simulink model "baseline_queso"  (R2021a)
settings: Solver=FixedStepAuto  StartTime=0.0  StopTime=10.0  FixedStep=framePeriod_s  RelTol=1e-3
undefined symbols (not defined in the file or in its folder): FlightMode, framePeriod_s, Spaaro, ThrottleVelocityRange
libraries: pid_lib x14, simulink x2, sharedtransform x1
(part 1 of 2)
settings Model: Creator=brian  LastModifiedBy=vaughnweirens
settings SolverCC: AlgebraicLoopSolver=TrustRegion
settings OptimizationCC: DefaultParameterBehavior=Inlined  GainParamInheritBuiltInType=on  UseFloatMulNetSlope=on  DefaultUnderspecifiedDataType=single  InlineInvariantSignals=on  PassReuseOutputArgsAs=Individual arguments  ZeroExternalMemoryAtStartup=off  ZeroInternalMemoryAtStartup=off  NoFixptDivByZeroProtection=on  EfficientFloat2IntCast=on  LifeSpan=1  OptimizeBlockOrder=speed  DifferentSizesBufferReuse=on  EfficientTunableParamExpr=on
settings DebuggingCC: ParameterTunabilityLossMsg=error  SFMachineParentedDataDiag=warning
settings HardwareCC: ProdBitPerPointer=32  ProdBitPerSizeT=32  ProdBitPerPtrDiffT=32  ProdLargestAtomicInteger=Long  ProdLargestAtomicFloat=Double  ProdWordSize=32  ProdLongLongMode=on  ProdHWDeviceType=NXP->Cortex-M4
settings ModelReferenceCC: ModelReferenceNumInstancesAllowed=Single
settings SFSimCC: SimParseCustomCode=off  MATLABDynamicMemAlloc=off
settings RTWCC: SystemTargetFile=ert.tlc  GenCodeOnly=on  TemplateMakefile=ert_default_tmf  RTWVerbose=off  Toolchain=Microsoft Visual C++ 2019 v16.0 | nmake (64-bit Windows)  BuildConfiguration=Faster Runs  TargetLang=C++
settings CodeAppCC: ForceParamTrailComments=on  IgnoreCustomStorageClasses=off  OperatorAnnotations=on  SimulinkDataObjDesc=on  SFDataObjDesc=on  CustomSymbolStrGlobalVar=rt$N$M  CustomSymbolStrType=$N$M  CustomSymbolStrFcn=$N$M$F  CustomSymbolStrMacro=$N$M  InsertBlockDesc=on
settings ERTTargetCC: TargetLangStandard=C++03 (ISO)  IncludeMdlTerminateFcn=off  CombineSignalStateStructs=on  SuppressErrorStatus=on  SupportAbsoluteTime=off  CodeInterfacePackaging=C++ class  SupportNonFinite=off  SupportComplex=off  ERTHeaderFileRootName=autocode$E  ERTSourceFileRootName=autocode$E  InlinedParameterPlacement=NonHierarchical  RootIOFormat=Structure reference  ERTCustomFileTemplate=example_file_process.tlc  ERTFilePackagingFormat=Compact  ArrayContainerType=std::array

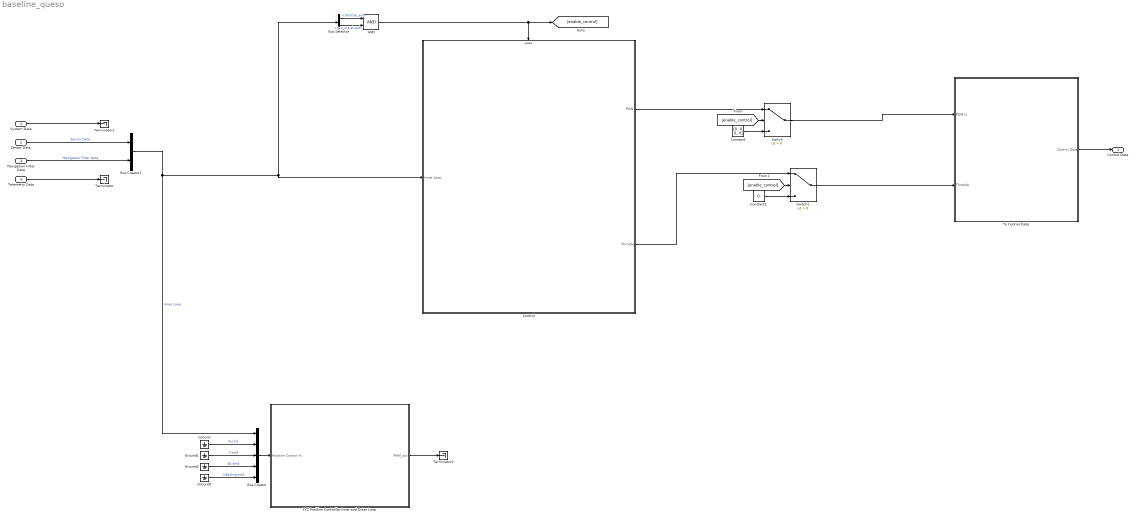
== system baseline_queso ==
  System Data : Inport  OutDataTypeStr=Bus: SysData  SampleTime=framePeriod_s  BusOutputAsStruct=on
  Sensor Data : Inport  Port=2  OutDataTypeStr=Bus: SensorData  SampleTime=framePeriod_s  BusOutputAsStruct=on
  Navigation Filter Data : Inport  Port=3  OutDataTypeStr=Bus: NavData  SampleTime=framePeriod_s  BusOutputAsStruct=on
  Telemetry Data : Inport  Port=4  OutDataTypeStr=Bus: TelemData  SampleTime=framePeriod_s  BusOutputAsStruct=on
  AND : Logic  IconShape=distinctive  AllPortsSameDT=off  OutDataTypeStr=boolean
  Bus Creator : BusCreator  Inputs=5
  Bus Creator1 : BusCreator  Inputs=2
  Bus Selector : BusSelector  OutputSignals=Sensor Data.inceptor.throttle_en,Navigation Filter Data.nav_initialized
  Constant : Constant  Value=[0, 0, 0, 0]  SampleTime=framePeriod_s
  Constant1 : Constant  Value=0  SampleTime=framePeriod_s
  Control : Subsystem
  Ground{,1..3} (4 alike) : Ground
  Switch : Switch  Criteria=u2 > Threshold
  Switch1 : Switch  Criteria=u2 > Threshold
  Terminator : Terminator
  Terminator1 : Terminator
  Terminator2 : Terminator
  To Control Data : Subsystem
  XYZ Position Controller Inner and Outer Loop : Subsystem
  Control Data : Outport  OutDataTypeStr=Bus: ControlData  SampleTime=framePeriod_s  BusOutputAsStruct=on
  wires:
  Telemetry Data/1 -> Terminator/1
  System Data/1 -> Terminator1/1
  Sensor Data/1 -> Bus Creator1/1  "Sensor Data"
  Navigation Filter Data/1 -> Bus Creator1/2  "Navigation Filter Data"
  Bus Creator1/1 -> Bus Creator/1, Bus Selector/1, Control/1(Inner Loop)  "Inner Loop"
  To Control Data/1(Control Data) -> Control Data/1
  Ground1/1 -> Bus Creator/3  "Y-cmd"
  Ground/1 -> Bus Creator/2  "X-cmd"
  Ground3/1 -> Bus Creator/5  "Heading-cmd"
  Ground2/1 -> Bus Creator/4  "Alt-cmd"
  Bus Creator/1 -> XYZ Position Controller Inner and Outer Loop/1(Position Control In)
  XYZ Position Controller Inner and Outer Loop/1(PWM_out) -> Terminator2/1
  Bus Selector/1 -> AND/1  "<throttle_en>"
  Bus Selector/2 -> AND/2  "<nav_initialized>"
  AND/1 -> [enable_control], Control/Enable
  [enable_control] -> Switch/2
  Constant/1 -> Switch/3
  Constant1/1 -> Switch1/3
  [enable_control] -> Switch1/2
  Control/1(PWM) -> Switch/1
  Control/2("Throttle ") -> Switch1/1
  Switch1/1 -> To Control Data/2("Throttle ")
  Switch/1 -> To Control Data/1(PWM In)

== system baseline_queso/Control ==
  Inner Loop : Inport
  Enable : EnablePort  PropagateVarSize=During execution
  Bus Creator4 : BusCreator  Inputs=4
  Inner Loop Control : Subsystem
  Motor Mixing Algorithm : Subsystem
  Outer Loop Control : Subsystem
  PWM : Outport
  "Throttle " : Outport  Port=2
  wires:
  Outer Loop Control/1("Throttle ") -> "Throttle "/1, Bus Creator4/1
  Motor Mixing Algorithm/1(PWM) -> PWM/1
  Inner Loop/1 -> Inner Loop Control/1(Inner Loop), Outer Loop Control/1(Outer Loop In)
  Inner Loop Control/3(Yaw) -> Bus Creator4/4
  Inner Loop Control/1(Roll) -> Bus Creator4/2
  Inner Loop Control/2(Pitch) -> Bus Creator4/3
  Bus Creator4/1 -> Motor Mixing Algorithm/1(MMA Bus)

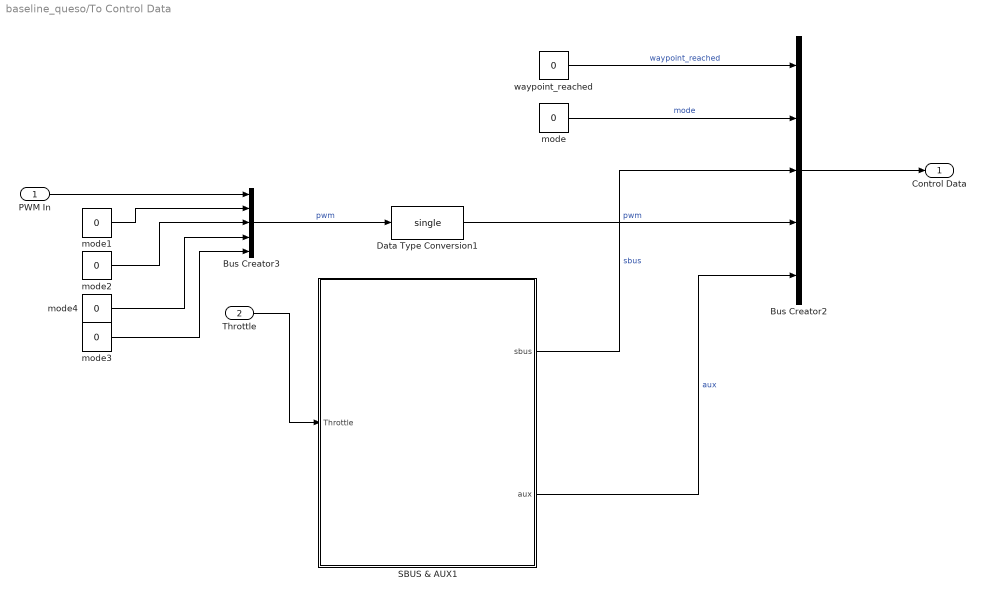
== system baseline_queso/To Control Data ==
  PWM In : Inport
  "Throttle " : Inport  Port=2
  Bus Creator2 : BusCreator  Inputs=5  OutDataTypeStr=Bus: ControlData  NonVirtualBus=on
  Bus Creator3 : BusCreator  Inputs=5
  Data Type Conversion1 : DataTypeConversion  OutDataTypeStr=single
  SBUS & AUX1 : Subsystem
  mode{,1..4} (5 alike) : Constant  Value=0  OutDataTypeStr=int8  SampleTime=framePeriod_s
  waypoint_reached : Constant  Value=0  OutDataTypeStr=boolean  SampleTime=framePeriod_s
  Control Data : Outport  OutDataTypeStr=Bus: ControlData  SampleTime=framePeriod_s  BusOutputAsStruct=on
  wires:
  waypoint_reached/1 -> Bus Creator2/1  "waypoint_reached"
  Bus Creator3/1 -> Data Type Conversion1/1  "pwm"
  mode/1 -> Bus Creator2/2  "mode"
  Bus Creator2/1 -> Control Data/1
  SBUS & AUX1/1(sbus) -> Bus Creator2/3  "sbus"
  SBUS & AUX1/2(aux) -> Bus Creator2/5  "aux"
  Data Type Conversion1/1 -> Bus Creator2/4  "pwm"
  PWM In/1 -> Bus Creator3/1
  "Throttle "/1 -> SBUS & AUX1/1("Throttle ")
  mode1/1 -> Bus Creator3/2
  mode2/1 -> Bus Creator3/3
  mode4/1 -> Bus Creator3/4
  mode3/1 -> Bus Creator3/5

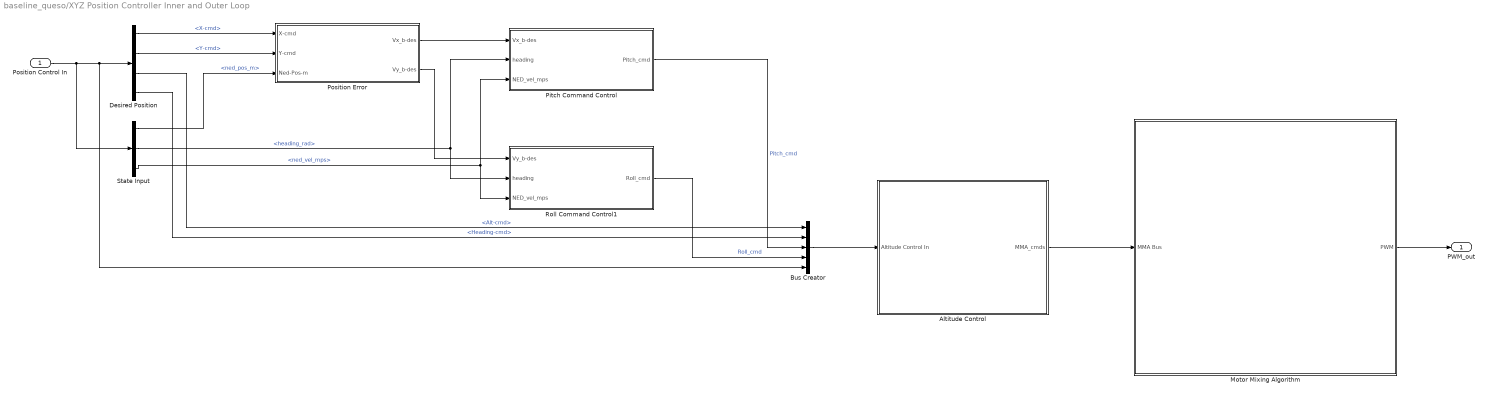
== system baseline_queso/XYZ Position Controller Inner and Outer Loop ==
  Position Control In : Inport
  Altitude Control : Subsystem
  Bus Creator : BusCreator  Inputs=5
  Desired Position : BusSelector  OutputSignals=X-cmd,Y-cmd,Alt-cmd,Heading-cmd
  Motor Mixing Algorithm : Subsystem
  Pitch Command Control : Subsystem
  Position Error : Subsystem
  Roll Command Control1 : Subsystem
  State Input : BusSelector  OutputSignals=Inner Loop.Navigation Filter Data.ned_pos_m,Inner Loop.Navigation Filter Data.heading_rad,Inner Loop.Navigation Filter Data.ned_vel_mps
  PWM_out : Outport
  wires:
  Position Control In/1 -> State Input/1, Bus Creator/5, Desired Position/1
  Desired Position/1 -> Position Error/1(X-cmd)  "<X-cmd>"
  Desired Position/2 -> Position Error/2(Y-cmd)  "<Y-cmd>"
  State Input/1 -> Position Error/3(Ned-Pos-m)  "<ned_pos_m>"
  Position Error/1(Vx_b-des) -> Pitch Command Control/1(Vx_b-des)
  State Input/3 -> Roll Command Control1/3(NED_vel_mps), Pitch Command Control/3(NED_vel_mps)  "<ned_vel_mps>"
  State Input/2 -> Pitch Command Control/2(heading), Roll Command Control1/2(heading)  "<heading_rad>"
  Position Error/2(Vy_b-des) -> Roll Command Control1/1(Vy_b-des)
  Bus Creator/1 -> Altitude Control/1(Altitude Control In)
  Desired Position/3 -> Bus Creator/1  "<Alt-cmd>"
  Desired Position/4 -> Bus Creator/2  "<Heading-cmd>"
  Pitch Command Control/1(Pitch_cmd) -> Bus Creator/3  "Pitch_cmd"
  Roll Command Control1/1(Roll_cmd) -> Bus Creator/4  "Roll_cmd"
  Altitude Control/1(MMA_cmds) -> Motor Mixing Algorithm/1(MMA Bus)
  Motor Mixing Algorithm/1(PWM) -> PWM_out/1

== system baseline_queso/Control/Inner Loop Control ==
  Inner Loop : Inport
  Pitch Controller : Subsystem
  Roll Controller : Subsystem
  Yaw Rate Controller : Subsystem
  Roll : Outport
  Pitch : Outport  Port=2
  Yaw : Outport  Port=3
  wires:
  Inner Loop/1 -> Yaw Rate Controller/1(Yaw Bus), Roll Controller/1(Roll Bus), Pitch Controller/1(Pitch Bus)
  Roll Controller/1(roll_cc) -> Roll/1  "roll_cc"
  Pitch Controller/1(pitch_cc) -> Pitch/1  "pitch_cc"
  Yaw Rate Controller/1(yaw_cc) -> Yaw/1  "yaw_cc"

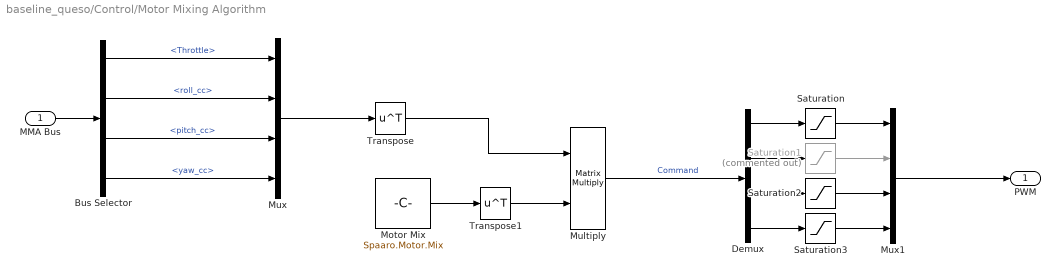
== system baseline_queso/Control/Motor Mixing Algorithm ==
  MMA Bus : Inport
  Bus Selector : BusSelector  OutputSignals=Throttle,roll_cc,pitch_cc,yaw_cc
  Demux : Demux
  Motor Mix : Constant  Value=Spaaro.Motor.Mix  OutDataTypeStr=single
  Multiply : Product  Inputs=**  Multiplication=Matrix(*)
  Mux : Mux
  Mux1 : Mux
  Saturation : Saturate  UpperLimit=1  LowerLimit=0
  Saturation1 : Saturate  Commented=on  UpperLimit=1  LowerLimit=0
  Saturation2 : Saturate  UpperLimit=1  LowerLimit=0
  Saturation3 : Saturate  UpperLimit=1  LowerLimit=0
  Transpose : Math  Operator=transpose  SaturateOnIntegerOverflow=on
  Transpose1 : Math  Operator=transpose  SaturateOnIntegerOverflow=on
  PWM : Outport
  wires:
  Mux/1 -> Transpose/1
  Transpose/1 -> Multiply/1
  Multiply/1 -> Demux/1  "Command"
  Saturation/1 -> Mux1/1
  Saturation1/1 -> Mux1/2
  Saturation2/1 -> Mux1/3
  Saturation3/1 -> Mux1/4
  Mux1/1 -> PWM/1
  Demux/1 -> Saturation/1
  Demux/2 -> Saturation1/1
  Demux/3 -> Saturation2/1
  Demux/4 -> Saturation3/1
  Motor Mix/1 -> Transpose1/1
  Transpose1/1 -> Multiply/2
  MMA Bus/1 -> Bus Selector/1
  Bus Selector/1 -> Mux/1  "<Throttle>"
  Bus Selector/2 -> Mux/2  "<roll_cc>"
  Bus Selector/3 -> Mux/3  "<pitch_cc>"
  Bus Selector/4 -> Mux/4  "<yaw_cc>"

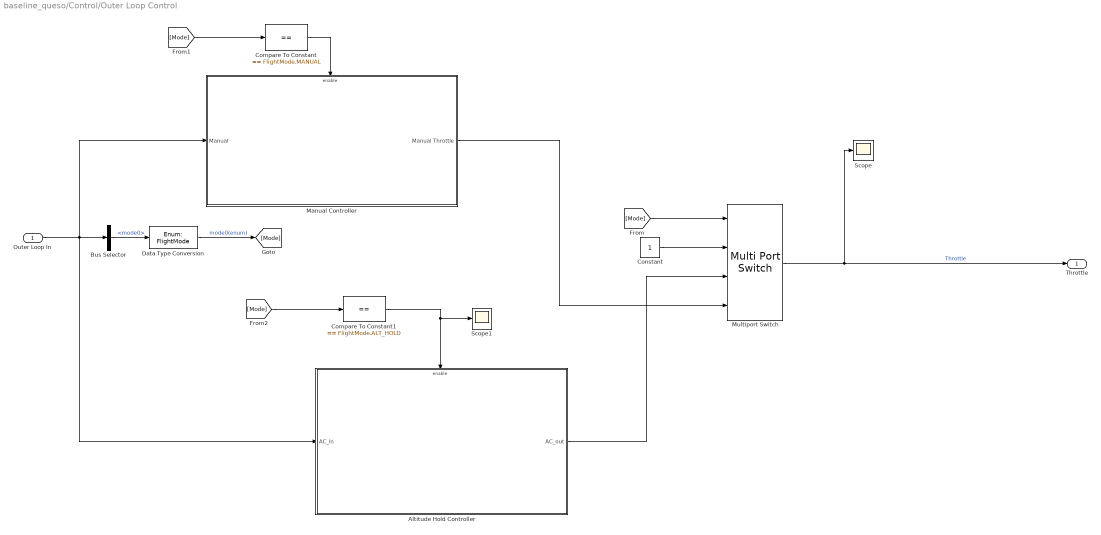
== system baseline_queso/Control/Outer Loop Control ==
  Outer Loop In : Inport
  Altitude Hold Controller : Subsystem
  Bus Selector : BusSelector  OutputSignals=Sensor Data.inceptor.mode0
  Compare To Constant : simulink/Logic and Bit Operations/Compare To Constant  relop===  const=FlightMode.MANUAL  OutDataTypeStr=boolean
  Compare To Constant1 : simulink/Logic and Bit Operations/Compare To Constant  relop===  const=FlightMode.ALT_HOLD  OutDataTypeStr=boolean
  Constant : Constant
  Data Type Conversion : DataTypeConversion  OutDataTypeStr=Enum: FlightMode
  Manual Controller : Subsystem
  Multiport Switch : MultiPortSwitch  DataPortOrder=Specify indices  DataPortIndices={FlightMode.AUTO, FlightMode.ALT_HOLD, FlightMode.MANUAL}
  Scope : Scope
  Scope1 : Scope
  "Throttle " : Outport
  wires:
  Multiport Switch/1 -> Scope/1, "Throttle "/1  "Throttle"
  [Mode] -> Compare To Constant/1
  Compare To Constant1/1 -> Scope1/1, Altitude Hold Controller/Enable
  Altitude Hold Controller/1(AC_out) -> Multiport Switch/3
  Compare To Constant/1 -> Manual Controller/Enable
  Data Type Conversion/1 -> [Mode]  "mode0(enum)"
  [Mode] -> Compare To Constant1/1
  [Mode] -> Multiport Switch/1
  Bus Selector/1 -> Data Type Conversion/1  "<mode0>"
  Outer Loop In/1 -> Altitude Hold Controller/1(AC_in), Bus Selector/1, Manual Controller/1(Manual)
  Constant/1 -> Multiport Switch/2
  Manual Controller/1(Manual Throttle) -> Multiport Switch/4

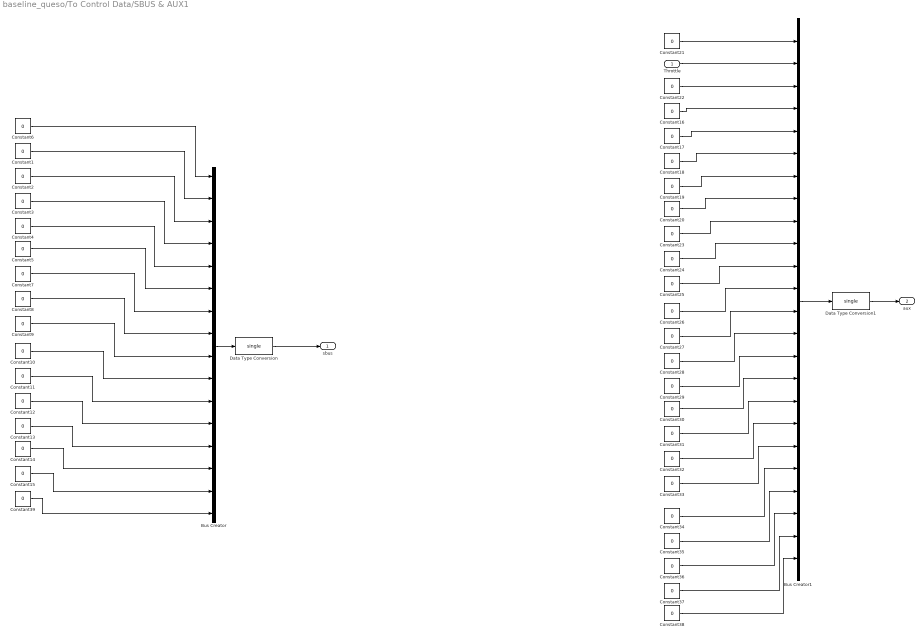
== system baseline_queso/To Control Data/SBUS & AUX1 ==
  "Throttle " : Inport
  Bus Creator : BusCreator  Inputs=16
  Bus Creator1 : BusCreator  Inputs=24
  Constant{1..39} (39 alike) : Constant  Value=0  OutDataTypeStr=single  SampleTime=framePeriod_s
  Data Type Conversion : DataTypeConversion  OutDataTypeStr=single
  Data Type Conversion1 : DataTypeConversion  OutDataTypeStr=single
  sbus : Outport  SampleTime=framePeriod_s
  aux : Outport  Port=2
  wires:
  Bus Creator/1 -> Data Type Conversion/1
  Data Type Conversion/1 -> sbus/1
  Bus Creator1/1 -> Data Type Conversion1/1
  Data Type Conversion1/1 -> aux/1
  Constant21/1 -> Bus Creator1/1
  "Throttle "/1 -> Bus Creator1/2
  Constant22/1 -> Bus Creator1/3
  Constant16/1 -> Bus Creator1/4
  Constant17/1 -> Bus Creator1/5
  Constant18/1 -> Bus Creator1/6
  Constant19/1 -> Bus Creator1/7
  Constant20/1 -> Bus Creator1/8
  Constant23/1 -> Bus Creator1/9
  Constant24/1 -> Bus Creator1/10
  Constant25/1 -> Bus Creator1/11
  Constant26/1 -> Bus Creator1/12
  Constant27/1 -> Bus Creator1/13
  Constant28/1 -> Bus Creator1/14
  Constant29/1 -> Bus Creator1/15
  Constant30/1 -> Bus Creator1/16
  Constant31/1 -> Bus Creator1/17
  Constant32/1 -> Bus Creator1/18
  Constant33/1 -> Bus Creator1/19
  Constant34/1 -> Bus Creator1/20
  Constant35/1 -> Bus Creator1/21
  Constant36/1 -> Bus Creator1/22
  Constant37/1 -> Bus Creator1/23
  Constant38/1 -> Bus Creator1/24
  Constant12/1 -> Bus Creator/12
  Constant11/1 -> Bus Creator/11
  Constant10/1 -> Bus Creator/10
  Constant9/1 -> Bus Creator/9
  Constant8/1 -> Bus Creator/8
  Constant7/1 -> Bus Creator/7
  Constant4/1 -> Bus Creator/5
  Constant5/1 -> Bus Creator/6
  Constant3/1 -> Bus Creator/4
  Constant2/1 -> Bus Creator/3
  Constant1/1 -> Bus Creator/2
  Constant6/1 -> Bus Creator/1
  Constant39/1 -> Bus Creator/16
  Constant15/1 -> Bus Creator/15
  Constant13/1 -> Bus Creator/13
  Constant14/1 -> Bus Creator/14

== system baseline_queso/XYZ Position Controller Inner and Outer Loop/Altitude Control ==
  Altitude Control In : Inport
  Bus Creator : BusCreator  Inputs=4
  Pitch Control : Subsystem
  Roll Control : Subsystem
  Throttle Control : Subsystem
  Yaw Control : Subsystem
  MMA_cmds : Outport
  wires:
  Altitude Control In/1 -> Throttle Control/1(Altitude Control In), Roll Control/1(Roll Control In), Pitch Control/1(Pitch Control In), Yaw Control/1(Yaw Control In)
  Bus Creator/1 -> MMA_cmds/1
  Throttle Control/1(Throttle_des) -> Bus Creator/1  "Throttle_des"
  Roll Control/1(Roll_cntrl) -> Bus Creator/2  "Roll_cntrl"
  Pitch Control/1(Pitch_cntrl) -> Bus Creator/3  "Pitch_cntrl"
  Yaw Control/1(Yaw_cntl) -> Bus Creator/4  "Yaw_cntrl"

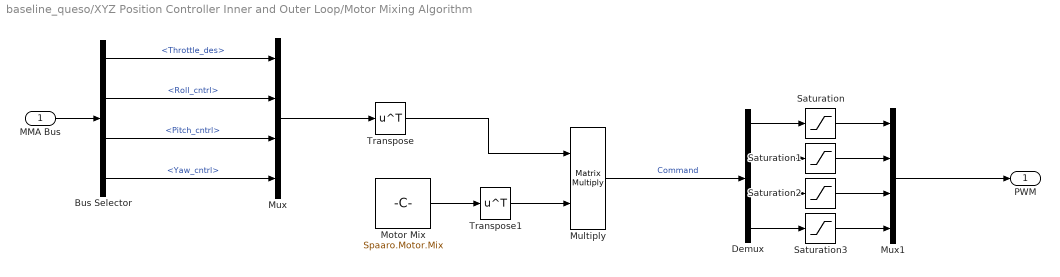
== system baseline_queso/XYZ Position Controller Inner and Outer Loop/Motor Mixing Algorithm ==
  MMA Bus : Inport
  Bus Selector : BusSelector  OutputSignals=Throttle_des,Roll_cntrl,Pitch_cntrl,Yaw_cntrl
  Demux : Demux
  Motor Mix : Constant  Value=Spaaro.Motor.Mix  OutDataTypeStr=single
  Multiply : Product  Inputs=**  Multiplication=Matrix(*)
  Mux : Mux
  Mux1 : Mux
  Saturation{,1..3} (4 alike) : Saturate  UpperLimit=1  LowerLimit=0
  Transpose : Math  Operator=transpose  SaturateOnIntegerOverflow=on
  Transpose1 : Math  Operator=transpose  SaturateOnIntegerOverflow=on
  PWM : Outport
  wires:
  Mux/1 -> Transpose/1
  Transpose/1 -> Multiply/1
  Multiply/1 -> Demux/1  "Command"
  Saturation/1 -> Mux1/1
  Saturation1/1 -> Mux1/2
  Saturation2/1 -> Mux1/3
  Saturation3/1 -> Mux1/4
  Mux1/1 -> PWM/1
  Demux/1 -> Saturation/1
  Demux/2 -> Saturation1/1
  Demux/3 -> Saturation2/1
  Demux/4 -> Saturation3/1
  Motor Mix/1 -> Transpose1/1
  Transpose1/1 -> Multiply/2
  MMA Bus/1 -> Bus Selector/1
  Bus Selector/1 -> Mux/1  "<Throttle_des>"
  Bus Selector/2 -> Mux/2  "<Roll_cntrl>"
  Bus Selector/3 -> Mux/3  "<Pitch_cntrl>"
  Bus Selector/4 -> Mux/4  "<Yaw_cntrl>"

== system baseline_queso/XYZ Position Controller Inner and Outer Loop/Pitch Command Control ==
  Vx_b-des : Inport
  heading : Inport  Port=2
  NED_vel_mps : Inport  Port=3
  Cos : Trigonometry  Operator=cos
  Divide : Product  Inputs=**
  PID Controller : pid_lib/PID Controller  Controller=PID  Form=Parallel  TimeDomain=Discrete-time  UseExternalTs=off  SampleTime=-1  IntegratorMethod=Forward Euler  FilterMethod=Forward Euler  ControllerParametersSource=internal  P=1  I=1  D=0  UseFilter=on  N=100  TunerSelectOption=Transfer Function Based (PID Tuner App)  InitialConditionSource=internal  InitialConditionForIntegrator=0  InitialConditionForFilter=0  DifferentiatorICPrevScaledInput=0  ExternalReset=none  TrackingMode=off  Kt=1  LimitOutput=off  SatLimitsSource=internal  UpperSaturationLimit=inf  LowerSaturationLimit=-inf  LinearizeAsGain=on  AntiWindupMode=none  Kb=1  POutMin=[]  POutMax=[]  IOutMin=[]  IOutMax=[]  DOutMin=[]  DOutMax=[]  NOutMin=[]  NOutMax=[]  SumOutMin=[]  SumOutMax=[]  SaturationOutMin=[]  SaturationOutMax=[]  PParamMin=[]  PParamMax=[]  IParamMin=[]  IParamMax=[]  DParamMin=[]  DParamMax=[]  NParamMin=[]  NParamMax=[]  KbParamMin=[]  KbParamMax=[]  KtParamMin=[]  KtParamMax=[]  KbOutMin=[]  KbOutMax=[]  KtOutMin=[]  KtOutMax=[]  IntegratorOutMin=[]  IntegratorOutMax=[]  FilterOutMin=[]  FilterOutMax=[]  SumI1OutMin=[]  SumI1OutMax=[]  SumI2OutMin=[]  SumI2OutMax=[]  SumI3OutMin=[]  SumI3OutMax=[]  SumI4OutMin=[]  SumI4OutMax=[]  SumDOutMin=[]  SumDOutMax=[]  DifferentiatorOutMin=[]  DifferentiatorOutMax=[]  FilterDiffOutCoefMin=[]  FilterDiffOutCoefMax=[]  ReciprocalOutMin=[]  ReciprocalOutMax=[]  SumDenOutMin=[]  SumDenOutMax=[]  SumNumOutMin=[]  SumNumOutMax=[]  DivideOutMin=[]  DivideOutMax=[]  UdiffTsProdOutMin=[]  UdiffTsProdOutMax=[]  NTsProdOutMin=[]  NTsProdOutMax=[]  UintegralTsProdOutMin=[]  UintegralTsProdOutMax=[]  UngainTsProdOutMin=[]  UngainTsProdOutMax=[]  IntegratorContinuousStateAttributes=''  IntegratorStateMustResolveToSignalObject=off  IntegratorRTWStateStorageClass=Auto  FilterContinuousStateAttributes=''  FilterStateMustResolveToSignalObject=off  FilterRTWStateStorageClass=Auto  ParallelPVariant=InternalParameters  IdealPVariant=Disabled  IVariant=InternalParameters  DVariant=InternalParameters  IntegratorVariant=Discrete  SatVariant=Disabled  AWVariant=Passthrough  PCopyVariant=Disabled  TRVariant=Disabled  FdbkBlocksVariant=Forward  IdealPFdbkVariant=Disabled  SatFdbkVariant=Disabled  DerivativeFilterVariant=ForwardEulerFilter  NVariant=InternalParameters  NCopyVariant=Disabled  FilterICVariant=InternalICsFilter  IntegratorICVariant=InternalICs  ExternalResetVariant=Disabled  TRSumVariant=Passthrough  SumFdbkVariant=Disabled  SumVariant=Sum_PID  TsampFilterVariant=InternalTs  TsampNgainVariant=Passthrough  TsampIntegralVariant=Passthrough  ExternalSaturationOutDataTypeStr=Inherit: Same as second input
  Selector : Selector  InputPortWidth=3  IndexOptions=Index vector (dialog)  Indices=[1]  OutputSizes=1
  Sum : Sum  Inputs=|+-
  Pitch_cmd : Outport
  wires:
  Vx_b-des/1 -> Sum/1
  heading/1 -> Cos/1
  NED_vel_mps/1 -> Selector/1
  Cos/1 -> Divide/1
  Selector/1 -> Divide/2
  Divide/1 -> Sum/2
  Sum/1 -> PID Controller/1
  PID Controller/1 -> Pitch_cmd/1

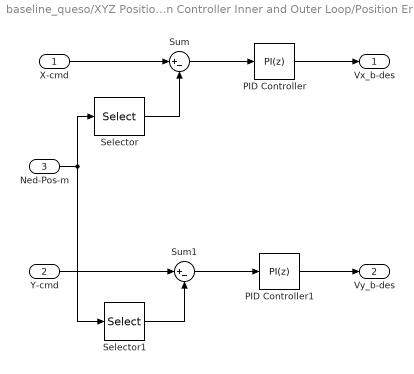
== system baseline_queso/XYZ Position Controller Inner and Outer Loop/Position Error ==
  X-cmd : Inport
  Y-cmd : Inport  Port=2
  Ned-Pos-m : Inport  Port=3
  PID Controller : pid_lib/PID Controller  Controller=PI  Form=Parallel  TimeDomain=Discrete-time  UseExternalTs=off  SampleTime=-1  IntegratorMethod=Forward Euler  FilterMethod=Forward Euler  ControllerParametersSource=internal  P=1  I=1  D=0  UseFilter=on  N=100  TunerSelectOption=Transfer Function Based (PID Tuner App)  InitialConditionSource=internal  InitialConditionForIntegrator=0  InitialConditionForFilter=0  DifferentiatorICPrevScaledInput=0  ExternalReset=none  TrackingMode=off  Kt=1  LimitOutput=off  SatLimitsSource=internal  UpperSaturationLimit=inf  LowerSaturationLimit=-inf  LinearizeAsGain=on  AntiWindupMode=none  Kb=1  POutMin=[]  POutMax=[]  IOutMin=[]  IOutMax=[]  DOutMin=[]  DOutMax=[]  NOutMin=[]  NOutMax=[]  SumOutMin=[]  SumOutMax=[]  SaturationOutMin=[]  SaturationOutMax=[]  PParamMin=[]  PParamMax=[]  IParamMin=[]  IParamMax=[]  DParamMin=[]  DParamMax=[]  NParamMin=[]  NParamMax=[]  KbParamMin=[]  KbParamMax=[]  KtParamMin=[]  KtParamMax=[]  KbOutMin=[]  KbOutMax=[]  KtOutMin=[]  KtOutMax=[]  IntegratorOutMin=[]  IntegratorOutMax=[]  FilterOutMin=[]  FilterOutMax=[]  SumI1OutMin=[]  SumI1OutMax=[]  SumI2OutMin=[]  SumI2OutMax=[]  SumI3OutMin=[]  SumI3OutMax=[]  SumI4OutMin=[]  SumI4OutMax=[]  SumDOutMin=[]  SumDOutMax=[]  DifferentiatorOutMin=[]  DifferentiatorOutMax=[]  FilterDiffOutCoefMin=[]  FilterDiffOutCoefMax=[]  ReciprocalOutMin=[]  ReciprocalOutMax=[]  SumDenOutMin=[]  SumDenOutMax=[]  SumNumOutMin=[]  SumNumOutMax=[]  DivideOutMin=[]  DivideOutMax=[]  UdiffTsProdOutMin=[]  UdiffTsProdOutMax=[]  NTsProdOutMin=[]  NTsProdOutMax=[]  UintegralTsProdOutMin=[]  UintegralTsProdOutMax=[]  UngainTsProdOutMin=[]  UngainTsProdOutMax=[]  IntegratorContinuousStateAttributes=''  IntegratorStateMustResolveToSignalObject=off  IntegratorRTWStateStorageClass=Auto  FilterContinuousStateAttributes=''  FilterStateMustResolveToSignalObject=off  FilterRTWStateStorageClass=Auto  ParallelPVariant=InternalParameters  IdealPVariant=Disabled  IVariant=InternalParameters  DVariant=Disabled  IntegratorVariant=Discrete  SatVariant=Disabled  AWVariant=Passthrough  PCopyVariant=Disabled  TRVariant=Disabled  FdbkBlocksVariant=Forward  IdealPFdbkVariant=Disabled  SatFdbkVariant=Disabled  DerivativeFilterVariant=Disabled  NVariant=Disabled  NCopyVariant=Disabled_SignalSpec  FilterICVariant=Disabled  IntegratorICVariant=InternalICs  ExternalResetVariant=Disabled  TRSumVariant=Passthrough  SumFdbkVariant=Disabled  SumVariant=Sum_PI  TsampFilterVariant=InternalTs  TsampNgainVariant=Passthrough  TsampIntegralVariant=Passthrough  ExternalSaturationOutDataTypeStr=Inherit: Same as second input
  PID Controller1 : pid_lib/PID Controller  Controller=PI  Form=Parallel  TimeDomain=Discrete-time  UseExternalTs=off  SampleTime=-1  IntegratorMethod=Forward Euler  FilterMethod=Forward Euler  ControllerParametersSource=internal  P=1  I=1  D=0  UseFilter=on  N=100  TunerSelectOption=Transfer Function Based (PID Tuner App)  InitialConditionSource=internal  InitialConditionForIntegrator=0  InitialConditionForFilter=0  DifferentiatorICPrevScaledInput=0  ExternalReset=none  TrackingMode=off  Kt=1  LimitOutput=off  SatLimitsSource=internal  UpperSaturationLimit=inf  LowerSaturationLimit=-inf  LinearizeAsGain=on  AntiWindupMode=none  Kb=1  POutMin=[]  POutMax=[]  IOutMin=[]  IOutMax=[]  DOutMin=[]  DOutMax=[]  NOutMin=[]  NOutMax=[]  SumOutMin=[]  SumOutMax=[]  SaturationOutMin=[]  SaturationOutMax=[]  PParamMin=[]  PParamMax=[]  IParamMin=[]  IParamMax=[]  DParamMin=[]  DParamMax=[]  NParamMin=[]  NParamMax=[]  KbParamMin=[]  KbParamMax=[]  KtParamMin=[]  KtParamMax=[]  KbOutMin=[]  KbOutMax=[]  KtOutMin=[]  KtOutMax=[]  IntegratorOutMin=[]  IntegratorOutMax=[]  FilterOutMin=[]  FilterOutMax=[]  SumI1OutMin=[]  SumI1OutMax=[]  SumI2OutMin=[]  SumI2OutMax=[]  SumI3OutMin=[]  SumI3OutMax=[]  SumI4OutMin=[]  SumI4OutMax=[]  SumDOutMin=[]  SumDOutMax=[]  DifferentiatorOutMin=[]  DifferentiatorOutMax=[]  FilterDiffOutCoefMin=[]  FilterDiffOutCoefMax=[]  ReciprocalOutMin=[]  ReciprocalOutMax=[]  SumDenOutMin=[]  SumDenOutMax=[]  SumNumOutMin=[]  SumNumOutMax=[]  DivideOutMin=[]  DivideOutMax=[]  UdiffTsProdOutMin=[]  UdiffTsProdOutMax=[]  NTsProdOutMin=[]  NTsProdOutMax=[]  UintegralTsProdOutMin=[]  UintegralTsProdOutMax=[]  UngainTsProdOutMin=[]  UngainTsProdOutMax=[]  IntegratorContinuousStateAttributes=''  IntegratorStateMustResolveToSignalObject=off  IntegratorRTWStateStorageClass=Auto  FilterContinuousStateAttributes=''  FilterStateMustResolveToSignalObject=off  FilterRTWStateStorageClass=Auto  ParallelPVariant=InternalParameters  IdealPVariant=Disabled  IVariant=InternalParameters  DVariant=Disabled  IntegratorVariant=Discrete  SatVariant=Disabled  AWVariant=Passthrough  PCopyVariant=Disabled  TRVariant=Disabled  FdbkBlocksVariant=Forward  IdealPFdbkVariant=Disabled  SatFdbkVariant=Disabled  DerivativeFilterVariant=Disabled  NVariant=Disabled  NCopyVariant=Disabled_SignalSpec  FilterICVariant=Disabled  IntegratorICVariant=InternalICs  ExternalResetVariant=Disabled  TRSumVariant=Passthrough  SumFdbkVariant=Disabled  SumVariant=Sum_PI  TsampFilterVariant=InternalTs  TsampNgainVariant=Passthrough  TsampIntegralVariant=Passthrough  ExternalSaturationOutDataTypeStr=Inherit: Same as second input
  Selector : Selector  InputPortWidth=3  IndexOptions=Index vector (dialog)  Indices=[1]  OutputSizes=1
  Selector1 : Selector  InputPortWidth=3  IndexOptions=Index vector (dialog)  Indices=[2]  OutputSizes=1
  Sum : Sum  Inputs=|+-
  Sum1 : Sum  Inputs=|+-
  Vx_b-des : Outport
  Vy_b-des : Outport  Port=2
  wires:
  X-cmd/1 -> Sum/1
  Y-cmd/1 -> Sum1/1
  Ned-Pos-m/1 -> Selector1/1, Selector/1
  Selector/1 -> Sum/2
  Selector1/1 -> Sum1/2
  Sum/1 -> PID Controller/1
  PID Controller/1 -> Vx_b-des/1
  Sum1/1 -> PID Controller1/1
  PID Controller1/1 -> Vy_b-des/1

== system baseline_queso/XYZ Position Controller Inner and Outer Loop/Roll Command Control1 ==
  Vy_b-des : Inport
  heading : Inport  Port=2
  NED_vel_mps : Inport  Port=3
  Cos : Trigonometry
  Divide : Product  Inputs=**
  PID Controller : pid_lib/PID Controller  Controller=PID  Form=Parallel  TimeDomain=Discrete-time  UseExternalTs=off  SampleTime=-1  IntegratorMethod=Forward Euler  FilterMethod=Forward Euler  ControllerParametersSource=internal  P=1  I=1  D=0  UseFilter=on  N=100  TunerSelectOption=Transfer Function Based (PID Tuner App)  InitialConditionSource=internal  InitialConditionForIntegrator=0  InitialConditionForFilter=0  DifferentiatorICPrevScaledInput=0  ExternalReset=none  TrackingMode=off  Kt=1  LimitOutput=off  SatLimitsSource=internal  UpperSaturationLimit=inf  LowerSaturationLimit=-inf  LinearizeAsGain=on  AntiWindupMode=none  Kb=1  POutMin=[]  POutMax=[]  IOutMin=[]  IOutMax=[]  DOutMin=[]  DOutMax=[]  NOutMin=[]  NOutMax=[]  SumOutMin=[]  SumOutMax=[]  SaturationOutMin=[]  SaturationOutMax=[]  PParamMin=[]  PParamMax=[]  IParamMin=[]  IParamMax=[]  DParamMin=[]  DParamMax=[]  NParamMin=[]  NParamMax=[]  KbParamMin=[]  KbParamMax=[]  KtParamMin=[]  KtParamMax=[]  KbOutMin=[]  KbOutMax=[]  KtOutMin=[]  KtOutMax=[]  IntegratorOutMin=[]  IntegratorOutMax=[]  FilterOutMin=[]  FilterOutMax=[]  SumI1OutMin=[]  SumI1OutMax=[]  SumI2OutMin=[]  SumI2OutMax=[]  SumI3OutMin=[]  SumI3OutMax=[]  SumI4OutMin=[]  SumI4OutMax=[]  SumDOutMin=[]  SumDOutMax=[]  DifferentiatorOutMin=[]  DifferentiatorOutMax=[]  FilterDiffOutCoefMin=[]  FilterDiffOutCoefMax=[]  ReciprocalOutMin=[]  ReciprocalOutMax=[]  SumDenOutMin=[]  SumDenOutMax=[]  SumNumOutMin=[]  SumNumOutMax=[]  DivideOutMin=[]  DivideOutMax=[]  UdiffTsProdOutMin=[]  UdiffTsProdOutMax=[]  NTsProdOutMin=[]  NTsProdOutMax=[]  UintegralTsProdOutMin=[]  UintegralTsProdOutMax=[]  UngainTsProdOutMin=[]  UngainTsProdOutMax=[]  IntegratorContinuousStateAttributes=''  IntegratorStateMustResolveToSignalObject=off  IntegratorRTWStateStorageClass=Auto  FilterContinuousStateAttributes=''  FilterStateMustResolveToSignalObject=off  FilterRTWStateStorageClass=Auto  ParallelPVariant=InternalParameters  IdealPVariant=Disabled  IVariant=InternalParameters  DVariant=InternalParameters  IntegratorVariant=Discrete  SatVariant=Disabled  AWVariant=Passthrough  PCopyVariant=Disabled  TRVariant=Disabled  FdbkBlocksVariant=Forward  IdealPFdbkVariant=Disabled  SatFdbkVariant=Disabled  DerivativeFilterVariant=ForwardEulerFilter  NVariant=InternalParameters  NCopyVariant=Disabled  FilterICVariant=InternalICsFilter  IntegratorICVariant=InternalICs  ExternalResetVariant=Disabled  TRSumVariant=Passthrough  SumFdbkVariant=Disabled  SumVariant=Sum_PID  TsampFilterVariant=InternalTs  TsampNgainVariant=Passthrough  TsampIntegralVariant=Passthrough  ExternalSaturationOutDataTypeStr=Inherit: Same as second input
  Selector : Selector  InputPortWidth=3  IndexOptions=Index vector (dialog)  Indices=[2]  OutputSizes=1
  Sum : Sum  Inputs=|+-
  Roll_cmd : Outport
  wires:
  Vy_b-des/1 -> Sum/1
  heading/1 -> Cos/1
  NED_vel_mps/1 -> Selector/1
  Cos/1 -> Divide/1
  Selector/1 -> Divide/2
  Divide/1 -> Sum/2
  Sum/1 -> PID Controller/1
  PID Controller/1 -> Roll_cmd/1

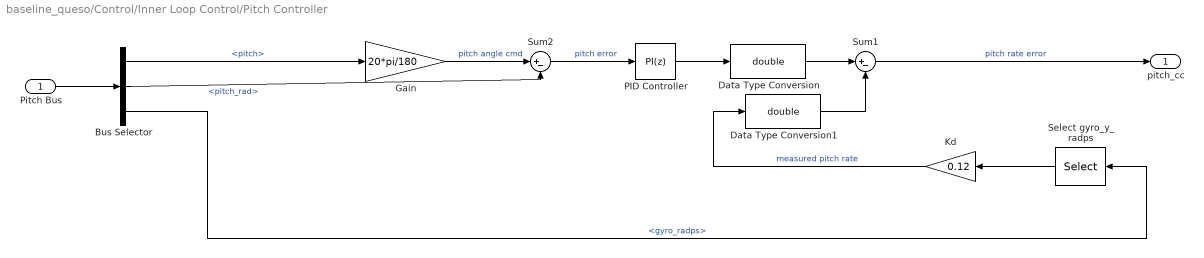
== system baseline_queso/Control/Inner Loop Control/Pitch Controller ==
  Pitch Bus : Inport
  Bus Selector : BusSelector  OutputSignals=Sensor Data.inceptor.pitch,Navigation Filter Data.pitch_rad,Navigation Filter Data.gyro_radps
  Data Type Conversion : DataTypeConversion  OutDataTypeStr=double
  Data Type Conversion1 : DataTypeConversion  OutDataTypeStr=double
  Gain : Gain  Gain=20*pi/180
  Kd : Gain  Gain=0.12
  PID Controller : pid_lib/PID Controller  Controller=PI  Form=Parallel  TimeDomain=Discrete-time  UseExternalTs=off  SampleTime=-1  IntegratorMethod=Forward Euler  FilterMethod=Forward Euler  ControllerParametersSource=internal  P=0.335  I=0.005  D=0  UseFilter=on  N=100  TunerSelectOption=Transfer Function Based (PID Tuner App)  InitialConditionSource=internal  InitialConditionForIntegrator=0  InitialConditionForFilter=0  DifferentiatorICPrevScaledInput=0  ExternalReset=none  TrackingMode=off  Kt=1  LimitOutput=on  SatLimitsSource=internal  UpperSaturationLimit=45*(pi/180)  LowerSaturationLimit=-45*(pi/180)  LinearizeAsGain=off  AntiWindupMode=clamping  Kb=1  POutMin=[]  POutMax=[]  IOutMin=[]  IOutMax=[]  DOutMin=[]  DOutMax=[]  NOutMin=[]  NOutMax=[]  SumOutMin=[]  SumOutMax=[]  SaturationOutMin=[]  SaturationOutMax=[]  PParamMin=[]  PParamMax=[]  IParamMin=[]  IParamMax=[]  DParamMin=[]  DParamMax=[]  NParamMin=[]  NParamMax=[]  KbParamMin=[]  KbParamMax=[]  KtParamMin=[]  KtParamMax=[]  KbOutMin=[]  KbOutMax=[]  KtOutMin=[]  KtOutMax=[]  IntegratorOutMin=[]  IntegratorOutMax=[]  FilterOutMin=[]  FilterOutMax=[]  SumI1OutMin=[]  SumI1OutMax=[]  SumI2OutMin=[]  SumI2OutMax=[]  SumI3OutMin=[]  SumI3OutMax=[]  SumI4OutMin=[]  SumI4OutMax=[]  SumDOutMin=[]  SumDOutMax=[]  DifferentiatorOutMin=[]  DifferentiatorOutMax=[]  FilterDiffOutCoefMin=[]  FilterDiffOutCoefMax=[]  ReciprocalOutMin=[]  ReciprocalOutMax=[]  SumDenOutMin=[]  SumDenOutMax=[]  SumNumOutMin=[]  SumNumOutMax=[]  DivideOutMin=[]  DivideOutMax=[]  UdiffTsProdOutMin=[]  UdiffTsProdOutMax=[]  NTsProdOutMin=[]  NTsProdOutMax=[]  UintegralTsProdOutMin=[]  UintegralTsProdOutMax=[]  UngainTsProdOutMin=[]  UngainTsProdOutMax=[]  IntegratorContinuousStateAttributes=''  IntegratorStateMustResolveToSignalObject=off  IntegratorRTWStateStorageClass=Auto  FilterContinuousStateAttributes=''  FilterStateMustResolveToSignalObject=off  FilterRTWStateStorageClass=Auto  ParallelPVariant=InternalParameters  IdealPVariant=Disabled  IVariant=InternalParameters  DVariant=Disabled  IntegratorVariant=Discrete  SatVariant=Enabled  AWVariant=DiscClampingParallel  PCopyVariant=Disabled  TRVariant=Disabled  FdbkBlocksVariant=Forward  IdealPFdbkVariant=Disabled  SatFdbkVariant=Disabled  DerivativeFilterVariant=Disabled  NVariant=Disabled  NCopyVariant=Disabled_SignalSpec  FilterICVariant=Disabled  IntegratorICVariant=InternalICs  ExternalResetVariant=Disabled  TRSumVariant=Passthrough  SumFdbkVariant=Disabled  SumVariant=Sum_PI  TsampFilterVariant=InternalTs  TsampNgainVariant=Passthrough  TsampIntegralVariant=Passthrough  ExternalSaturationOutDataTypeStr=Inherit: Same as second input
  Select gyro_y_radps : Selector  InputPortWidth=3  IndexOptions=Index vector (dialog)  Indices=[2]  OutputSizes=1
  Sum1 : Sum  Inputs=|+-
  Sum2 : Sum  Inputs=|+-
  pitch_cc : Outport
  wires:
  Gain/1 -> Sum2/1  "pitch angle cmd"
  Kd/1 -> Data Type Conversion1/1  "measured pitch rate"
  Sum1/1 -> pitch_cc/1  "pitch rate error"
  Sum2/1 -> PID Controller/1  "pitch error"
  Select gyro_y_radps/1 -> Kd/1
  PID Controller/1 -> Data Type Conversion/1
  Pitch Bus/1 -> Bus Selector/1
  Bus Selector/1 -> Gain/1  "<pitch>"
  Bus Selector/2 -> Sum2/2  "<pitch_rad>"
  Bus Selector/3 -> Select gyro_y_radps/1  "<gyro_radps>"
  Data Type Conversion/1 -> Sum1/1
  Data Type Conversion1/1 -> Sum1/2

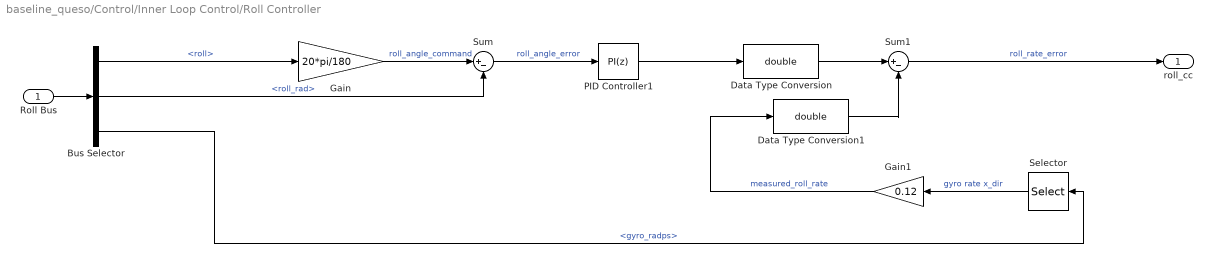
== system baseline_queso/Control/Inner Loop Control/Roll Controller ==
  Roll Bus : Inport
  Bus Selector : BusSelector  OutputSignals=Sensor Data.inceptor.roll,Navigation Filter Data.roll_rad,Navigation Filter Data.gyro_radps
  Data Type Conversion : DataTypeConversion  OutDataTypeStr=double
  Data Type Conversion1 : DataTypeConversion  OutDataTypeStr=double
  Gain : Gain  Gain=20*pi/180
  Gain1 : Gain  Gain=0.12
  PID Controller1 : pid_lib/PID Controller  Controller=PI  Form=Parallel  TimeDomain=Discrete-time  UseExternalTs=off  SampleTime=-1  IntegratorMethod=Forward Euler  FilterMethod=Forward Euler  ControllerParametersSource=internal  P=0.335  I=0.005  D=0  UseFilter=on  N=100  TunerSelectOption=Transfer Function Based (PID Tuner App)  InitialConditionSource=internal  InitialConditionForIntegrator=0  InitialConditionForFilter=0  DifferentiatorICPrevScaledInput=0  ExternalReset=none  TrackingMode=off  Kt=1  LimitOutput=on  SatLimitsSource=internal  UpperSaturationLimit=45*(pi/180)  LowerSaturationLimit=-45*(pi/180)  LinearizeAsGain=off  AntiWindupMode=clamping  Kb=1  POutMin=[]  POutMax=[]  IOutMin=[]  IOutMax=[]  DOutMin=[]  DOutMax=[]  NOutMin=[]  NOutMax=[]  SumOutMin=[]  SumOutMax=[]  SaturationOutMin=[]  SaturationOutMax=[]  PParamMin=[]  PParamMax=[]  IParamMin=[]  IParamMax=[]  DParamMin=[]  DParamMax=[]  NParamMin=[]  NParamMax=[]  KbParamMin=[]  KbParamMax=[]  KtParamMin=[]  KtParamMax=[]  KbOutMin=[]  KbOutMax=[]  KtOutMin=[]  KtOutMax=[]  IntegratorOutMin=[]  IntegratorOutMax=[]  FilterOutMin=[]  FilterOutMax=[]  SumI1OutMin=[]  SumI1OutMax=[]  SumI2OutMin=[]  SumI2OutMax=[]  SumI3OutMin=[]  SumI3OutMax=[]  SumI4OutMin=[]  SumI4OutMax=[]  SumDOutMin=[]  SumDOutMax=[]  DifferentiatorOutMin=[]  DifferentiatorOutMax=[]  FilterDiffOutCoefMin=[]  FilterDiffOutCoefMax=[]  ReciprocalOutMin=[]  ReciprocalOutMax=[]  SumDenOutMin=[]  SumDenOutMax=[]  SumNumOutMin=[]  SumNumOutMax=[]  DivideOutMin=[]  DivideOutMax=[]  UdiffTsProdOutMin=[]  UdiffTsProdOutMax=[]  NTsProdOutMin=[]  NTsProdOutMax=[]  UintegralTsProdOutMin=[]  UintegralTsProdOutMax=[]  UngainTsProdOutMin=[]  UngainTsProdOutMax=[]  IntegratorContinuousStateAttributes=''  IntegratorStateMustResolveToSignalObject=off  IntegratorRTWStateStorageClass=Auto  FilterContinuousStateAttributes=''  FilterStateMustResolveToSignalObject=off  FilterRTWStateStorageClass=Auto  ParallelPVariant=InternalParameters  IdealPVariant=Disabled  IVariant=InternalParameters  DVariant=Disabled  IntegratorVariant=Discrete  SatVariant=Enabled  AWVariant=DiscClampingParallel  PCopyVariant=Disabled  TRVariant=Disabled  FdbkBlocksVariant=Forward  IdealPFdbkVariant=Disabled  SatFdbkVariant=Disabled  DerivativeFilterVariant=Disabled  NVariant=Disabled  NCopyVariant=Disabled_SignalSpec  FilterICVariant=Disabled  IntegratorICVariant=InternalICs  ExternalResetVariant=Disabled  TRSumVariant=Passthrough  SumFdbkVariant=Disabled  SumVariant=Sum_PI  TsampFilterVariant=InternalTs  TsampNgainVariant=Passthrough  TsampIntegralVariant=Passthrough  ExternalSaturationOutDataTypeStr=Inherit: Same as second input
  Selector : Selector  InputPortWidth=3  IndexOptions=Index vector (dialog)  Indices=[1]  OutputSizes=1
  Sum : Sum  Inputs=|+-
  Sum1 : Sum  Inputs=|+-
  roll_cc : Outport
  wires:
  Sum1/1 -> roll_cc/1  "roll_rate_error"
  Gain/1 -> Sum/1  "roll_angle_command"
  Gain1/1 -> Data Type Conversion1/1  "measured_roll_rate"
  Sum/1 -> PID Controller1/1  "roll_angle_error"
  Selector/1 -> Gain1/1  "gyro rate x_dir"
  PID Controller1/1 -> Data Type Conversion/1
  Roll Bus/1 -> Bus Selector/1
  Bus Selector/1 -> Gain/1  "<roll>"
  Bus Selector/2 -> Sum/2  "<roll_rad>"
  Bus Selector/3 -> Selector/1  "<gyro_radps>"
  Data Type Conversion/1 -> Sum1/1
  Data Type Conversion1/1 -> Sum1/2

== system baseline_queso/Control/Inner Loop Control/Yaw Rate Controller ==
  Yaw Bus : Inport
  Bus Selector : BusSelector  OutputSignals=Sensor Data.inceptor.yaw,Navigation Filter Data.gyro_radps
  Data Type Conversion : DataTypeConversion  OutDataTypeStr=double
  PID Controller : pid_lib/PID Controller  Controller=PI  Form=Parallel  TimeDomain=Discrete-time  UseExternalTs=off  SampleTime=-1  IntegratorMethod=Forward Euler  FilterMethod=Forward Euler  ControllerParametersSource=internal  P=1.85  I=0.01  D=0  UseFilter=on  N=100  TunerSelectOption=Transfer Function Based (PID Tuner App)  InitialConditionSource=internal  InitialConditionForIntegrator=0  InitialConditionForFilter=0  DifferentiatorICPrevScaledInput=0  ExternalReset=none  TrackingMode=off  Kt=1  LimitOutput=on  SatLimitsSource=internal  UpperSaturationLimit=90*pi/180  LowerSaturationLimit=-90*pi/180  LinearizeAsGain=off  AntiWindupMode=clamping  Kb=1  POutMin=[]  POutMax=[]  IOutMin=[]  IOutMax=[]  DOutMin=[]  DOutMax=[]  NOutMin=[]  NOutMax=[]  SumOutMin=[]  SumOutMax=[]  SaturationOutMin=[]  SaturationOutMax=[]  PParamMin=[]  PParamMax=[]  IParamMin=[]  IParamMax=[]  DParamMin=[]  DParamMax=[]  NParamMin=[]  NParamMax=[]  KbParamMin=[]  KbParamMax=[]  KtParamMin=[]  KtParamMax=[]  KbOutMin=[]  KbOutMax=[]  KtOutMin=[]  KtOutMax=[]  IntegratorOutMin=[]  IntegratorOutMax=[]  FilterOutMin=[]  FilterOutMax=[]  SumI1OutMin=[]  SumI1OutMax=[]  SumI2OutMin=[]  SumI2OutMax=[]  SumI3OutMin=[]  SumI3OutMax=[]  SumI4OutMin=[]  SumI4OutMax=[]  SumDOutMin=[]  SumDOutMax=[]  DifferentiatorOutMin=[]  DifferentiatorOutMax=[]  FilterDiffOutCoefMin=[]  FilterDiffOutCoefMax=[]  ReciprocalOutMin=[]  ReciprocalOutMax=[]  SumDenOutMin=[]  SumDenOutMax=[]  SumNumOutMin=[]  SumNumOutMax=[]  DivideOutMin=[]  DivideOutMax=[]  UdiffTsProdOutMin=[]  UdiffTsProdOutMax=[]  NTsProdOutMin=[]  NTsProdOutMax=[]  UintegralTsProdOutMin=[]  UintegralTsProdOutMax=[]  UngainTsProdOutMin=[]  UngainTsProdOutMax=[]  IntegratorContinuousStateAttributes=''  IntegratorStateMustResolveToSignalObject=off  IntegratorRTWStateStorageClass=Auto  FilterContinuousStateAttributes=''  FilterStateMustResolveToSignalObject=off  FilterRTWStateStorageClass=Auto  ParallelPVariant=InternalParameters  IdealPVariant=Disabled  IVariant=InternalParameters  DVariant=Disabled  IntegratorVariant=Discrete  SatVariant=Enabled  AWVariant=DiscClampingParallel  PCopyVariant=Disabled  TRVariant=Disabled  FdbkBlocksVariant=Forward  IdealPFdbkVariant=Disabled  SatFdbkVariant=Disabled  DerivativeFilterVariant=Disabled  NVariant=Disabled  NCopyVariant=Disabled_SignalSpec  FilterICVariant=Disabled  IntegratorICVariant=InternalICs  ExternalResetVariant=Disabled  TRSumVariant=Passthrough  SumFdbkVariant=Disabled  SumVariant=Sum_PI  TsampFilterVariant=InternalTs  TsampNgainVariant=Passthrough  TsampIntegralVariant=Passthrough  ExternalSaturationOutDataTypeStr=Inherit: Same as second input
  Saturation Gain : Gain  Gain=20*(pi/180)
  Selector : Selector  InputPortWidth=3  IndexOptions=Index vector (dialog)  Indices=3  OutputSizes=1
  Sum1 : Sum  Inputs=|+-
  yaw_cc : Outport
  wires:
  Yaw Bus/1 -> Bus Selector/1
  Saturation Gain/1 -> Sum1/1
  Sum1/1 -> Data Type Conversion/1
  Selector/1 -> Sum1/2
  PID Controller/1 -> yaw_cc/1
  Bus Selector/1 -> Saturation Gain/1  "<yaw>"
  Bus Selector/2 -> Selector/1  "<gyro_radps>"
  Data Type Conversion/1 -> PID Controller/1

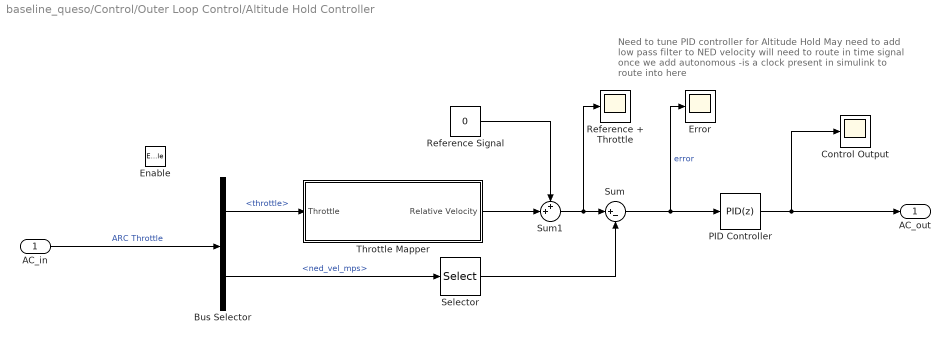
== system baseline_queso/Control/Outer Loop Control/Altitude Hold Controller ==
  note: Need to tune PID controller for Altitude Hold
      | May need to add low pass filter to NED velocity
      | will need to route in time signal once we add autonomous
      | -is a clock present in simulink to route into here
  AC_in : Inport
  Enable : EnablePort  PropagateVarSize=During execution
  Bus Selector : BusSelector  OutputSignals=Sensor Data.inceptor.throttle,Navigation Filter Data.ned_vel_mps
  Control Output : Scope
  Error : Scope
  PID Controller : pid_lib/PID Controller  Controller=PID  Form=Parallel  TimeDomain=Discrete-time  UseExternalTs=off  SampleTime=framePeriod_s  IntegratorMethod=Forward Euler  FilterMethod=Forward Euler  ControllerParametersSource=internal  P=0  I=0  D=0  UseFilter=on  N=100  TunerSelectOption=Frequency Response Based  InitialConditionSource=internal  InitialConditionForIntegrator=0  InitialConditionForFilter=0  DifferentiatorICPrevScaledInput=0  ExternalReset=none  TrackingMode=off  Kt=1  LimitOutput=off  SatLimitsSource=internal  UpperSaturationLimit=inf  LowerSaturationLimit=-inf  LinearizeAsGain=on  AntiWindupMode=none  Kb=1  POutMin=[]  POutMax=[]  IOutMin=[]  IOutMax=[]  DOutMin=[]  DOutMax=[]  NOutMin=[]  NOutMax=[]  SumOutMin=[]  SumOutMax=[]  SaturationOutMin=[]  SaturationOutMax=[]  PParamMin=[]  PParamMax=[]  IParamMin=[]  IParamMax=[]  DParamMin=[]  DParamMax=[]  NParamMin=[]  NParamMax=[]  KbParamMin=[]  KbParamMax=[]  KtParamMin=[]  KtParamMax=[]  KbOutMin=[]  KbOutMax=[]  KtOutMin=[]  KtOutMax=[]  IntegratorOutMin=[]  IntegratorOutMax=[]  FilterOutMin=[]  FilterOutMax=[]  SumI1OutMin=[]  SumI1OutMax=[]  SumI2OutMin=[]  SumI2OutMax=[]  SumI3OutMin=[]  SumI3OutMax=[]  SumI4OutMin=[]  SumI4OutMax=[]  SumDOutMin=[]  SumDOutMax=[]  DifferentiatorOutMin=[]  DifferentiatorOutMax=[]  FilterDiffOutCoefMin=[]  FilterDiffOutCoefMax=[]  ReciprocalOutMin=[]  ReciprocalOutMax=[]  SumDenOutMin=[]  SumDenOutMax=[]  SumNumOutMin=[]  SumNumOutMax=[]  DivideOutMin=[]  DivideOutMax=[]  UdiffTsProdOutMin=[]  UdiffTsProdOutMax=[]  NTsProdOutMin=[]  NTsProdOutMax=[]  UintegralTsProdOutMin=[]  UintegralTsProdOutMax=[]  UngainTsProdOutMin=[]  UngainTsProdOutMax=[]  IntegratorContinuousStateAttributes=''  IntegratorStateMustResolveToSignalObject=off  IntegratorRTWStateStorageClass=Auto  FilterContinuousStateAttributes=''  FilterStateMustResolveToSignalObject=off  FilterRTWStateStorageClass=Auto  ParallelPVariant=InternalParameters  IdealPVariant=Disabled  IVariant=InternalParameters  DVariant=InternalParameters  IntegratorVariant=Discrete  SatVariant=Disabled  AWVariant=Passthrough  PCopyVariant=Disabled  TRVariant=Disabled  FdbkBlocksVariant=Forward  IdealPFdbkVariant=Disabled  SatFdbkVariant=Disabled  DerivativeFilterVariant=ForwardEulerFilter  NVariant=InternalParameters  NCopyVariant=Disabled  FilterICVariant=InternalICsFilter  IntegratorICVariant=InternalICs  ExternalResetVariant=Disabled  TRSumVariant=Passthrough  SumFdbkVariant=Disabled  SumVariant=Sum_PID  TsampFilterVariant=InternalTs  TsampNgainVariant=Passthrough  TsampIntegralVariant=Passthrough  ExternalSaturationOutDataTypeStr=Inherit: Same as second input
  Reference + Throttle : Scope
  Reference Signal : Constant  Value=0  SampleTime=framePeriod_s
  Selector : Selector  InputPortWidth=3  IndexOptions=Index vector (dialog)  Indices=[3]  OutputSizes=1
  Sum : Sum  Inputs=|+-
  Sum1 : Sum  Inputs=++|
  Throttle Mapper : Subsystem
  AC_out : Outport  SampleTime=framePeriod_s
  wires:
  AC_in/1 -> Bus Selector/1  "ARC Throttle"
  Bus Selector/1 -> Throttle Mapper/1(Throttle)  "<throttle>"
  Bus Selector/2 -> Selector/1  "<ned_vel_mps>"
  Selector/1 -> Sum/2
  Sum/1 -> PID Controller/1, Error/1  "error"
  Sum1/1 -> Reference + Throttle/1, Sum/1
  Reference Signal/1 -> Sum1/1
  Throttle Mapper/1(Relative Velocity) -> Sum1/2
  PID Controller/1 -> Control Output/1, AC_out/1

== system baseline_queso/Control/Outer Loop Control/Manual Controller ==
  Manual : Inport
  Enable : EnablePort  PropagateVarSize=During execution
  Bus Selector : BusSelector  OutputSignals=Sensor Data.inceptor.throttle
  Manual Throttle : Outport
  wires:
  Manual/1 -> Bus Selector/1
  Bus Selector/1 -> Manual Throttle/1  "<throttle>"

== system baseline_queso/XYZ Position Controller Inner and Outer Loop/Altitude Control/Pitch Control ==
  Pitch Control In : Inport
  Bus Selector : BusSelector  OutputSignals=Pitch_cmd,signal5.Inner Loop.Navigation Filter Data.pitch_rad,signal5.Inner Loop.Navigation Filter Data.gyro_bias_radps
  Data Type Conversion : DataTypeConversion  OutDataTypeStr=double
  Kd : Gain  Gain=0.12
  PID Controller : pid_lib/PID Controller  Controller=PI  Form=Parallel  TimeDomain=Discrete-time  UseExternalTs=off  SampleTime=-1  IntegratorMethod=Forward Euler  FilterMethod=Forward Euler  ControllerParametersSource=internal  P=0.335  I=0.005  D=0  UseFilter=on  N=100  TunerSelectOption=Transfer Function Based (PID Tuner App)  InitialConditionSource=internal  InitialConditionForIntegrator=0  InitialConditionForFilter=0  DifferentiatorICPrevScaledInput=0  ExternalReset=none  TrackingMode=off  Kt=1  LimitOutput=on  SatLimitsSource=internal  UpperSaturationLimit=45*(pi/180)  LowerSaturationLimit=-45*(pi/180)  LinearizeAsGain=off  AntiWindupMode=clamping  Kb=1  POutMin=[]  POutMax=[]  IOutMin=[]  IOutMax=[]  DOutMin=[]  DOutMax=[]  NOutMin=[]  NOutMax=[]  SumOutMin=[]  SumOutMax=[]  SaturationOutMin=[]  SaturationOutMax=[]  PParamMin=[]  PParamMax=[]  IParamMin=[]  IParamMax=[]  DParamMin=[]  DParamMax=[]  NParamMin=[]  NParamMax=[]  KbParamMin=[]  KbParamMax=[]  KtParamMin=[]  KtParamMax=[]  KbOutMin=[]  KbOutMax=[]  KtOutMin=[]  KtOutMax=[]  IntegratorOutMin=[]  IntegratorOutMax=[]  FilterOutMin=[]  FilterOutMax=[]  SumI1OutMin=[]  SumI1OutMax=[]  SumI2OutMin=[]  SumI2OutMax=[]  SumI3OutMin=[]  SumI3OutMax=[]  SumI4OutMin=[]  SumI4OutMax=[]  SumDOutMin=[]  SumDOutMax=[]  DifferentiatorOutMin=[]  DifferentiatorOutMax=[]  FilterDiffOutCoefMin=[]  FilterDiffOutCoefMax=[]  ReciprocalOutMin=[]  ReciprocalOutMax=[]  SumDenOutMin=[]  SumDenOutMax=[]  SumNumOutMin=[]  SumNumOutMax=[]  DivideOutMin=[]  DivideOutMax=[]  UdiffTsProdOutMin=[]  UdiffTsProdOutMax=[]  NTsProdOutMin=[]  NTsProdOutMax=[]  UintegralTsProdOutMin=[]  UintegralTsProdOutMax=[]  UngainTsProdOutMin=[]  UngainTsProdOutMax=[]  IntegratorContinuousStateAttributes=''  IntegratorStateMustResolveToSignalObject=off  IntegratorRTWStateStorageClass=Auto  FilterContinuousStateAttributes=''  FilterStateMustResolveToSignalObject=off  FilterRTWStateStorageClass=Auto  ParallelPVariant=InternalParameters  IdealPVariant=Disabled  IVariant=InternalParameters  DVariant=Disabled  IntegratorVariant=Discrete  SatVariant=Enabled  AWVariant=DiscClampingParallel  PCopyVariant=Disabled  TRVariant=Disabled  FdbkBlocksVariant=Forward  IdealPFdbkVariant=Disabled  SatFdbkVariant=Disabled  DerivativeFilterVariant=Disabled  NVariant=Disabled  NCopyVariant=Disabled_SignalSpec  FilterICVariant=Disabled  IntegratorICVariant=InternalICs  ExternalResetVariant=Disabled  TRSumVariant=Passthrough  SumFdbkVariant=Disabled  SumVariant=Sum_PI  TsampFilterVariant=InternalTs  TsampNgainVariant=Passthrough  TsampIntegralVariant=Passthrough  ExternalSaturationOutDataTypeStr=Inherit: Same as second input
  Select gyro_y_radps : Selector  InputPortWidth=3  IndexOptions=Index vector (dialog)  Indices=[2]  OutputSizes=1
  Sum1 : Sum  Inputs=|+-
  Sum2 : Sum  Inputs=|+-
  Pitch_cntrl : Outport
  wires:
  Kd/1 -> Sum1/2  "measured pitch rate"
  Bus Selector/3 -> Select gyro_y_radps/1  "<gyro_bias_radps>"
  PID Controller/1 -> Sum1/1
  Select gyro_y_radps/1 -> Kd/1
  Sum1/1 -> Data Type Conversion/1  "pitch rate error"
  Sum2/1 -> PID Controller/1  "pitch error"
  Pitch Control In/1 -> Bus Selector/1
  Bus Selector/1 -> Sum2/1  "<Pitch_cmd>"
  Bus Selector/2 -> Sum2/2  "<pitch_rad>"
  Data Type Conversion/1 -> Pitch_cntrl/1
